simulink model "Drone2_simulink_old1"  (R2024b)
settings: Solver=ode1be  StartTime=0.0  StopTime=1200  FixedStep=0.001  MaxStep=0.001  MinStep=0.00095  RelTol=1e-3
undefined symbols (not defined in the file): DiscIntNeverNeededParam, Environment, Newton, Raphson, Sim3dSensor, Vehicle, X, Y, Z
libraries: sm_lib x2951, nesl_utility x76, slpidlib x25, simulink x4, eeGeneralControl x4, matrix_library x3, rllib x2, sim3dlib x2, uavsim3dlib x2, dspstat3 x1, SignalEditorBlockLib x1, sharedutil x1
(part 5 of 21)

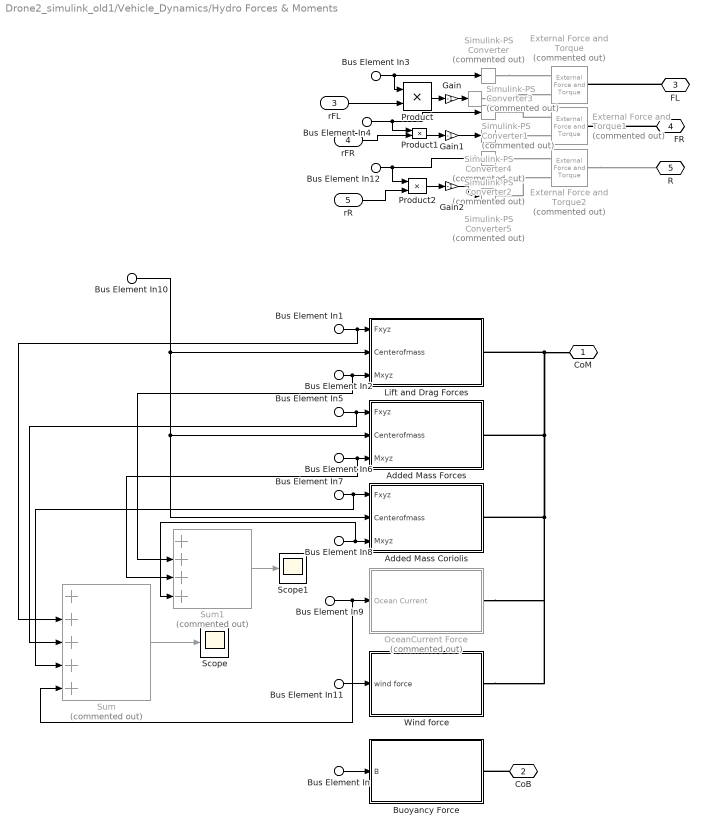
== system Drone2_simulink_old1/Vehicle_Dynamics/Hydro Forces & Moments ==
  Bus Element In1 : Inport  PortName=HydroForces  Element=Drag.Forces
  Bus Element In2 : Inport  PortName=HydroForces  Element=Drag.Moments
  Bus Element In : Inport  PortName=HydroForces  Element=BuoyancyForce
  Bus Element In5 : Inport  PortName=HydroForces  Element=AddedMass.AMForcesXYZ
  Bus Element In6 : Inport  PortName=HydroForces  Element=AddedMass.AMMomentsXYZ
  Bus Element In7 : Inport  PortName=HydroForces  Element=AddedMass.CForcesXYZ
  Bus Element In8 : Inport  PortName=HydroForces  Element=AddedMass.CMomentsXYZ
  Bus Element In9 : Inport  PortName=HydroForces  Element=OceanCurrentForce
  Bus Element In11 : Inport  PortName=HydroForces  Element=WindForce
  Bus Element In3 : Inport  PortName=HydroForces  Element=syringe.FL
  Bus Element In4 : Inport  PortName=HydroForces  Element=syringe.FR
  Bus Element In12 : Inport  PortName=HydroForces  Element=syringe.R
  Bus Element In10 : Inport  Port=2  PortName=CenterofMass  Element=Body.COM
  rFL : Inport  Port=3
  rFR : Inport  Port=4
  rR : Inport  Port=5
  Added Mass Coriolis : Subsystem
  Added Mass Forces : Subsystem
  Buoyancy Force : Subsystem
  External Force and Torque : sm_lib/Forces and Torques/External Force and Torque  Commented=on  EnableForceX=off  EnableForceY=off  EnableForceZ=on  EnableForce=off  ForceResolutionFrame=AttachedFrame  EnableTorqueX=off  EnableTorqueY=on  EnableTorqueZ=off  EnableTorque=off  TorqueResolutionFrame=AttachedFrame
  External Force and Torque1 : sm_lib/Forces and Torques/External Force and Torque  Commented=on  EnableForceX=off  EnableForceY=off  EnableForceZ=on  EnableForce=off  ForceResolutionFrame=AttachedFrame  EnableTorqueX=off  EnableTorqueY=on  EnableTorqueZ=off  EnableTorque=off  TorqueResolutionFrame=AttachedFrame
  External Force and Torque2 : sm_lib/Forces and Torques/External Force and Torque  Commented=on  EnableForceX=off  EnableForceY=off  EnableForceZ=on  EnableForce=off  ForceResolutionFrame=AttachedFrame  EnableTorqueX=off  EnableTorqueY=on  EnableTorqueZ=off  EnableTorque=off  TorqueResolutionFrame=AttachedFrame
  Gain : Gain  Gain=-1
  Gain1 : Gain  Gain=-1
  Gain2 : Gain  Gain=-1
  Lift and Drag Forces : Subsystem
  OceanCurrent Force : Subsystem  Commented=on
  Product : Product
  Product1 : Product
  Product2 : Product
  Scope : Scope
  Scope1 : Scope
  Simulink-PS Converter{,1..5} (6 alike) : nesl_utility/Simulink-PS Converter  Commented=on  PhysicalDomain=network_engine_domain  SubClassName=ps_input  LeftPortType=input  RightPortType=output  PseudoPeriodic=off  Frequencies=[]  NoiseDistribution=none  NoiseParameters=[]  Unit=1  AffineConversion=off  FilteringAndDerivatives=provide  SimscapeFilterOrder=1  InputFilterTimeConstant=0.001  UdotUserProvided=0
  Sum : Sum  Commented=on  Inputs=+++++
  Sum1 : Sum  Commented=on  Inputs=++++
  Wind force : Subsystem
  CoM : PMIOPort  Side=Left
  CoB : PMIOPort  Port=2  Side=Left
  FL : PMIOPort  Port=3  Side=Left
  FR : PMIOPort  Port=4  Side=Left
  R : PMIOPort  Port=5  Side=Left
  wires:
  Bus Element In/1 -> Buoyancy Force/1(B)
  Bus Element In1/1 -> Sum/2, Lift and Drag Forces/1(Fxyz)
  Bus Element In2/1 -> Sum1/2, Lift and Drag Forces/3(Mxyz)
  Bus Element In5/1 -> Sum/3, Added Mass Forces/1(Fxyz)
  Bus Element In8/1 -> Sum1/4, Added Mass Coriolis/3(Mxyz)
  Bus Element In9/1 -> Sum/5, OceanCurrent Force/1(Ocean Current)
  Bus Element In10/1 -> Lift and Drag Forces/2(Centerofmass), Added Mass Coriolis/2(Centerofmass), Added Mass Forces/2(Centerofmass)
  Bus Element In6/1 -> Sum1/3, Added Mass Forces/3(Mxyz)
  Bus Element In7/1 -> Sum/4, Added Mass Coriolis/1(Fxyz)
  Bus Element In11/1 -> Wind force/1(wind force)
  Sum/1 -> Scope/1
  Sum1/1 -> Scope1/1
  Bus Element In3/1 -> Product/1, Simulink-PS Converter/1
  Bus Element In4/1 -> Simulink-PS Converter1/1, Product1/1
  Product/1 -> Gain/1
  Gain1/1 -> Simulink-PS Converter4/1
  Gain2/1 -> Simulink-PS Converter5/1
  rFL/1 -> Product/2
  rFR/1 -> Product1/2
  Gain/1 -> Simulink-PS Converter3/1
  Product1/1 -> Gain1/1
  Bus Element In12/1 -> Product2/1, Simulink-PS Converter2/1
  rR/1 -> Product2/2
  Product2/1 -> Gain2/1
  connections:
  CoB/RConn1 -- Buoyancy Force/RConn1
  Wind force/RConn1 -- OceanCurrent Force/RConn1 -- Added Mass Coriolis/RConn1 -- Added Mass Forces/RConn1 -- CoM/RConn1 -- Lift and Drag Forces/RConn1
  Simulink-PS Converter/RConn1 -- External Force and Torque/LConn1
  External Force and Torque1/LConn1 -- Simulink-PS Converter1/RConn1
  Simulink-PS Converter2/RConn1 -- External Force and Torque2/LConn1
  FL/RConn1 -- External Force and Torque/RConn1
  FR/RConn1 -- External Force and Torque1/RConn1
  External Force and Torque2/RConn1 -- R/RConn1
  Simulink-PS Converter3/RConn1 -- External Force and Torque/LConn2
  Simulink-PS Converter4/RConn1 -- External Force and Torque1/LConn2
  Simulink-PS Converter5/RConn1 -- External Force and Torque2/LConn2

== system Drone2_simulink_old1/Vehicle_Dynamics/World ==
  Bottom floor : Subsystem  mask{ZB=-10, X=25, Z=0.1, Y=25, C1R=0.600, C1G=1, C1B=1.0, C2R=0, C2G=0.4, C2B=0.6}
      mask prompts: ZB "Distance of Bottom from World"; X "Length"; Z "Thikness"; Y "Width"; C1R "Red"; C1G "Green"; C1B "Blue"; C2R "Red"; C2G "Green"; C2B "Blue"
      mask init:
      | Color1 = [C1R C1G C1B];
      | Color2 = [C2R C2G C2B];
      mask DialogControl ParameterGroupVar Prompt: Bottom surface data
      mask DialogControl Container8 Prompt: Distance from World to Bottom
      mask DialogControl Container6 Prompt: Data of Each tiles
      mask DialogControl Container7 Prompt: Color 1
      mask DialogControl Container5 Prompt: Color2
      mask Display:
      | patch([0 10 10 0], [0 0 10 10], Color1);
      | patch([10 20 20 10], [0 0 10 10], Color2);
      | patch([0 10 10 0], [10 10 20 20], Color2);
      | patch([10 20 20 10], [10 10 20 20], Color1);
  Bottom floor1 : Subsystem  mask{ZB=-40, X=25, Z=0.1, Y=25, C1R=0.780, C1G=1.0, C1B=0.660, C2R=1.0, C2G=0.0, C2B=1.0}
      mask prompts: ZB "Distance of Bottom from World"; X "Length"; Z "Thikness"; Y "Width"; C1R "Red"; C1G "Green"; C1B "Blue"; C2R "Red"; C2G "Green"; C2B "Blue"
      mask init:
      | Color1 = [C1R C1G C1B];
      | Color2 = [C2R C2G C2B];
      mask DialogControl ParameterGroupVar Prompt: Bottom surface data
      mask DialogControl Container8 Prompt: Distance from World to Bottom
      mask DialogControl Container6 Prompt: Data of Each tiles
      mask DialogControl Container7 Prompt: Color 1
      mask DialogControl Container5 Prompt: Color2
      mask Display:
      | patch([0 10 10 0], [0 0 10 10], Color1);
      | patch([10 20 20 10], [0 0 10 10], Color2);
      | patch([0 10 10 0], [10 10 20 20], Color2);
      | patch([10 20 20 10], [10 10 20 20], Color1);
  Brick Solid : sm_lib/Body Elements/Brick Solid  Commented=on  BrickDimensions=[0.5 1 10]  BrickDimensionsUnits=m  ExportEntireGeometry=off  InertiaType=CalculateFromGeometry  BasedOnType=Density  Density=1000  DensityUnits=kg/m^3  Mass=1  MassUnits=kg  CenterOfMass=[0 0 0]  CenterOfMassUnits=m  MomentsOfInertia=[1 1 1]  MomentsOfInertiaUnits=kg*m^2  ProductsOfInertia=[0 0 0]  ProductsOfInertiaUnits=kg*m^2  GraphicType=FromGeometry  MarkerShape=Sphere  MarkerSize=10  GraphicVisPropType=SimpleVisualProperties  GraphicDiffuseColor=[1.0 0.2 0.2]  GraphicOpacity=1  GraphicSpecularColor=[0.5 0.5 0.5 1.0]  GraphicAmbientColor=[0.15 0.15 0.15 1.0]  GraphicEmissiveColor=[0.0 0.0 0.0 1.0]  GraphicShininess=75  DoExposeReferenceFrame=on  SerializedFrames=<Frames/>
  Brick Solid1 : sm_lib/Body Elements/Brick Solid  Commented=on  BrickDimensions=[0.5 1 10]  BrickDimensionsUnits=m  ExportEntireGeometry=off  InertiaType=CalculateFromGeometry  BasedOnType=Density  Density=1000  DensityUnits=kg/m^3  Mass=1  MassUnits=kg  CenterOfMass=[0 0 0]  CenterOfMassUnits=m  MomentsOfInertia=[1 1 1]  MomentsOfInertiaUnits=kg*m^2  ProductsOfInertia=[0 0 0]  ProductsOfInertiaUnits=kg*m^2  GraphicType=FromGeometry  MarkerShape=Sphere  MarkerSize=10  GraphicVisPropType=SimpleVisualProperties  GraphicDiffuseColor=[1.0 0.2 0.2]  GraphicOpacity=1  GraphicSpecularColor=[0.5 0.5 0.5 1.0]  GraphicAmbientColor=[0.15 0.15 0.15 1.0]  GraphicEmissiveColor=[0.0 0.0 0.0 1.0]  GraphicShininess=75  DoExposeReferenceFrame=on  SerializedFrames=<Frames/>
  MechanismConfiguration : sm_lib/Utilities/Mechanism Configuration  UniformGravity=Constant  GravityVector=[0 0 Environment.gravity]  GravityVectorUnits=m/s^2  LinearizationDelta=0.001  JointModeTransitionNonlinearIterations=2
  Solver Configuration : nesl_utility/Solver Configuration  PhysicalDomain=network_engine_domain  SubClassName=solver  LeftPortType=input  RightPortType=generic  Tones=[]  Harmonics=[]  SimulateNoise=off  Profile=off  UseLocalSampling=off  EnableSwitchedLinearOptims=on  FrequencyDomain=off  UseCCode=off  RelTol=0.001  AbsTol=0.001  MinStep=1e-09  ToWorkspace=off  RevertToSquareIcSolve=off  NumHomotopyIterations=100  PhasorMode=off  PhasorModeNumHarmonics=1  ConsistencySolver=NEWTON_XTOL_AFTER_FTOL  IndexReductionMethod=DerivativeReplacement  DoDC=off  ResidualTolerance=1e-09  ConsistencyTolSource=LOCAL  ConsistencyAbsTol=0.001  ConsistencyRelTol=0.001  ConsistencyTolFactor=0.001  UseLocalSolver=on  LocalSolverChoice=NE_BACKWARD_EULER_ADVANCER  ResolveIndetEquations=on  FunctionEvalNumThread=1  LocalSolverSampleTime=0.001  DoFixedCost=on  MaxNonlinIter=3  MaxModeIter=2  ComputeImpulses=off  ImpulseIterations=2  LinearAlgebra=Sparse  LinearAlgebraNumThread=0  EquationFormulation=NE_TIME_EF  DelaysMemoryBudget=1024  AutomaticFiltering=off  FilteringTimeConstant=0.001  PartitionStorageMethod=AS_NEEDED  PartitionMemoryBudget=1024  PartitionMethod=ROBUST  MultibodyUseLocalSolver=off  MultibodyLocalSolverChoice=ODE4  MultibodyLocalSolverSampleTime=0.001
  Spatial Contact Force : sm_lib/Forces and Torques/Spatial Contact Force  NormalForceType=SmoothSpringDamper  NormalStiffness=1  NormalStiffnessUnits=N/m  NormalDamping=0.001  NormalDampingUnits=N/(m/s)  NormalTransitionRegionWidth=0.05  NormalTransitionRegionWidthUnits=m  FrictionType=None  CoefficientOfStaticFriction=0  CoefficientOfDynamicFriction=0  FrictionalCriticalVelocity=1  FrictionalCriticalVelocityUnits=m/s  SenseContactSignal=off  SensePenetrationDepth=off  SenseSeparationDistance=off  SenseNormalForceMagnitude=off  SenseFrictionalForceMagnitude=off  SenseNormalVelocity=off  SenseTangentialVelocity=off  SenseContactBaseRotation=off  SenseContactBaseTranslation=off  SenseContactFollowerRotation=off  SenseContactFollowerTranslation=off  ZeroCrossDetectContactStartAndEnd=off
  Spatial Contact Force1 : sm_lib/Forces and Torques/Spatial Contact Force  NormalForceType=SmoothSpringDamper  NormalStiffness=1e2  NormalStiffnessUnits=N/m  NormalDamping=1e3  NormalDampingUnits=N/(m/s)  NormalTransitionRegionWidth=1e-4  NormalTransitionRegionWidthUnits=m  FrictionType=SmoothStickSlip  CoefficientOfStaticFriction=0.5  CoefficientOfDynamicFriction=0.3  FrictionalCriticalVelocity=1e-3  FrictionalCriticalVelocityUnits=m/s  SenseContactSignal=off  SensePenetrationDepth=off  SenseSeparationDistance=off  SenseNormalForceMagnitude=off  SenseFrictionalForceMagnitude=off  SenseNormalVelocity=off  SenseTangentialVelocity=off  SenseContactBaseRotation=off  SenseContactBaseTranslation=off  SenseContactFollowerRotation=off  SenseContactFollowerTranslation=off  ZeroCrossDetectContactStartAndEnd=off
  World : sm_lib/Frames and Transforms/World Frame
  water surface : sm_lib/Body Elements/Brick Solid  BrickDimensions=[500 500 0.01]  BrickDimensionsUnits=m  ExportEntireGeometry=on  InertiaType=CalculateFromGeometry  BasedOnType=Density  Density=1  DensityUnits=kg/m^3  Mass=1  MassUnits=kg  CenterOfMass=[0 0 0]  CenterOfMassUnits=m  MomentsOfInertia=[1 1 1]  MomentsOfInertiaUnits=kg*m^2  ProductsOfInertia=[0 0 0]  ProductsOfInertiaUnits=kg*m^2  GraphicType=FromGeometry  MarkerShape=Sphere  MarkerSize=10  GraphicVisPropType=SimpleVisualProperties  GraphicDiffuseColor=[0.0 0.8 1.0]  GraphicOpacity=0.1  GraphicSpecularColor=[0.5 0.5 0.5 1.0]  GraphicAmbientColor=[0.15 0.15 0.15 1.0]  GraphicEmissiveColor=[0.0 0.0 0.0 1.0]  GraphicShininess=75  DoExposeReferenceFrame=on  SerializedFrames=<Frames/>
  water surface ti bottom : sm_lib/Frames and Transforms/Rigid Transform  RotationMethod=None  FollAlignAxisA=+X  BaseAlignAxisA=+Y  FollAlignAxisB=+Y  BaseAlignAxisB=+Z  RotationStandardAxis=+Z  RotationAngle=0  RotationAngleUnits=deg  RotationArbitraryAxis=[0 0 1]  RotationSequenceAxes=FollowerAxes  RotationSequence=XYX  RotationSequenceAngles=[0 0 0]  RotationSequenceAnglesUnits=deg  RotationMatrix=[1 0 0;0 1 0;0 0 1]  Quaternion=[1 0 0 0]  TranslationMethod=Cartesian  TranslationCartesianOffset=[0 0 0]  TranslationCartesianOffsetUnits=m  TranslationStandardAxis=+Z  TranslationStandardOffset=0  TranslationStandardOffsetUnits=m  TranslationROffset=0  TranslationROffsetUnits=m  TranslationThetaOffset=0  TranslationThetaOffsetUnits=deg  TranslationZOffset=0  TranslationZOffsetUnits=m
  water surface ti bottom1 : sm_lib/Frames and Transforms/Rigid Transform  Commented=on  RotationMethod=None  FollAlignAxisA=+X  BaseAlignAxisA=+Y  FollAlignAxisB=+Y  BaseAlignAxisB=+Z  RotationStandardAxis=+Z  RotationAngle=0  RotationAngleUnits=deg  RotationArbitraryAxis=[0 0 1]  RotationSequenceAxes=FollowerAxes  RotationSequence=XYX  RotationSequenceAngles=[0 0 0]  RotationSequenceAnglesUnits=deg  RotationMatrix=[1 0 0;0 1 0;0 0 1]  Quaternion=[1 0 0 0]  TranslationMethod=Cartesian  TranslationCartesianOffset=[25 0 -5]  TranslationCartesianOffsetUnits=m  TranslationStandardAxis=+Z  TranslationStandardOffset=0  TranslationStandardOffsetUnits=m  TranslationROffset=0  TranslationROffsetUnits=m  TranslationThetaOffset=0  TranslationThetaOffsetUnits=deg  TranslationZOffset=0  TranslationZOffsetUnits=m
  water surface ti bottom2 : sm_lib/Frames and Transforms/Rigid Transform  Commented=on  RotationMethod=None  FollAlignAxisA=+X  BaseAlignAxisA=+Y  FollAlignAxisB=+Y  BaseAlignAxisB=+Z  RotationStandardAxis=+Z  RotationAngle=0  RotationAngleUnits=deg  RotationArbitraryAxis=[0 0 1]  RotationSequenceAxes=FollowerAxes  RotationSequence=XYX  RotationSequenceAngles=[0 0 0]  RotationSequenceAnglesUnits=deg  RotationMatrix=[1 0 0;0 1 0;0 0 1]  Quaternion=[1 0 0 0]  TranslationMethod=Cartesian  TranslationCartesianOffset=[10 15 -5]  TranslationCartesianOffsetUnits=m  TranslationStandardAxis=+Z  TranslationStandardOffset=0  TranslationStandardOffsetUnits=m  TranslationROffset=0  TranslationROffsetUnits=m  TranslationThetaOffset=0  TranslationThetaOffsetUnits=deg  TranslationZOffset=0  TranslationZOffsetUnits=m
  water surface ti bottom3 : sm_lib/Frames and Transforms/Rigid Transform  RotationMethod=AlignedAxes  FollAlignAxisA=+X  BaseAlignAxisA=+X  FollAlignAxisB=-Z  BaseAlignAxisB=+Y  RotationStandardAxis=+Z  RotationAngle=0  RotationAngleUnits=deg  RotationArbitraryAxis=[0 0 1]  RotationSequenceAxes=FollowerAxes  RotationSequence=XYX  RotationSequenceAngles=[0 0 0]  RotationSequenceAnglesUnits=deg  RotationMatrix=[1 0 0;0 1 0;0 0 1]  Quaternion=[1 0 0 0]  TranslationMethod=Cartesian  TranslationCartesianOffset=[0 0 0]  TranslationCartesianOffsetUnits=m  TranslationStandardAxis=+Z  TranslationStandardOffset=0  TranslationStandardOffsetUnits=m  TranslationROffset=0  TranslationROffsetUnits=m  TranslationThetaOffset=0  TranslationThetaOffsetUnits=deg  TranslationZOffset=0  TranslationZOffsetUnits=m
  surface : PMIOPort  Side=Right
  bottomsurf : PMIOPort  Port=2  Side=Right
  W : PMIOPort  Port=3  Side=Right
  connections:
  water surface/LConn1 -- Spatial Contact Force/LConn1
  surface/RConn1 -- Spatial Contact Force/RConn1
  bottomsurf/RConn1 -- Spatial Contact Force1/RConn1
  World/RConn1 -- water surface ti bottom3/LConn1 -- water surface ti bottom1/LConn1 -- water surface ti bottom2/LConn1 -- Solver Configuration/RConn1 -- water surface ti bottom/LConn1 -- water surface/RConn1 -- MechanismConfiguration/RConn1 -- W/RConn1
  Bottom floor/LConn1 -- water surface ti bottom/RConn1
  Bottom floor/RConn1 -- Spatial Contact Force1/LConn1
  Brick Solid/RConn1 -- water surface ti bottom1/RConn1
  Brick Solid1/RConn1 -- water surface ti bottom2/RConn1
  Bottom floor1/LConn1 -- water surface ti bottom3/RConn1

== system Drone2_simulink_old1/Visualization/psidot ==
  pqr : Inport
  phithetapsi : Inport  Port=2
  Mux1 : Mux  Inputs=[3 3 3]
  psidot : Fcn  Expr=(u[2]*u[4]+u[3]*u[7])/u[8]
  sincos : Trigonometry  Operator=sincos
  psid : Outport  Unit=rad/s  InitialOutput=0  VectorParamsAs1DForOutWhenUnconnected=off
  wires:
  sincos/2 -> Mux1/3
  sincos/1 -> Mux1/2
  phithetapsi/1 -> sincos/1
  pqr/1 -> Mux1/1
  Mux1/1 -> psidot/1
  psidot/1 -> psid/1

== system Drone2_simulink_old1/Controller (STA-Based)/Subsystem1/norm force ==
  force : Inport
  Add : Sum
  Add2 : Sum  Inputs=|++
  Demux2 : Demux  Outputs=2
  Gain : Gain  Gain=2
  Gain1 : Gain  Gain=2
  Sqrt : Sqrt
  Square : Math  Operator=square
  Square1 : Math  Operator=square
  Terminator : Terminator
  sum : Outport
  wires:
  Square1/1 -> Add/2
  Add/1 -> Sqrt/1
  Demux2/1 -> Gain1/1, Square/1
  Demux2/2 -> Add2/2, Square1/1
  Square/1 -> Gain/1
  force/1 -> Demux2/1
  Gain/1 -> Add/1
  Gain1/1 -> Add2/1
  Add2/1 -> sum/1
  Sqrt/1 -> Terminator/1  "norm"

== system Drone2_simulink_old1/Drive Controls/Thrust Controls/Depth and Pitch Control ==
  note: NOTE: Vehicle depth is indirectly controlled by the pitch angle which is regulated by the vertical thrusters ONLY
  PPf : Inport
  SPf : Inport  Port=2
  ZRef : Inport  Port=3
  Z : Inport  Port=4
  theta : Inport  Port=5
  Gain2 : Gain  Gain=-1
  Main Propellers Thrust Offset Compensation : Subsystem
  PDtheta : slpidlib/PID Controller  Controller=PD  Form=Parallel  TimeDomain=Continuous-time  UseExternalTs=off  SampleTime=-1  IntegratorMethod=Forward Euler  FilterMethod=Forward Euler  ControllerParametersSource=internal  P=-2023.58  I=1  UseKiTs=off  D=-2454.43  UseExternalDerivativeSource=off  N=3588.47  UseFilter=on  TunerSelectOption=Transfer Function Based (PID Tuner App)  InitialConditionSource=internal  InitialConditionForIntegrator=0  InitialConditionForFilter=0  DifferentiatorICPrevScaledInput=0  ExternalReset=none  TrackingMode=off  Kt=1  LimitOutput=off  SatLimitsSource=internal  UpperSaturationLimit=inf  LowerSaturationLimit=-inf  LinearizeAsGain=on  AntiWindupMode=none  Kb=1  LimitIntegrator=off  UpperIntegratorSaturationLimit=inf  LowerIntegratorSaturationLimit=-inf  POutMin=[]  POutMax=[]  IOutMin=[]  IOutMax=[]  DOutMin=[]  DOutMax=[]  NOutMin=[]  NOutMax=[]  SumOutMin=[]  SumOutMax=[]  SaturationOutMin=[]  SaturationOutMax=[]  PParamMin=[]  PParamMax=[]  IParamMin=[]  IParamMax=[]  DParamMin=[]  DParamMax=[]  NParamMin=[]  NParamMax=[]  KbParamMin=[]  KbParamMax=[]  KtParamMin=[]  KtParamMax=[]  KbOutMin=[]  KbOutMax=[]  KtOutMin=[]  KtOutMax=[]  IntegratorOutMin=[]  IntegratorOutMax=[]  FilterOutMin=[]  FilterOutMax=[]  SumI1OutMin=[]  SumI1OutMax=[]  SumI2OutMin=[]  SumI2OutMax=[]  SumI3OutMin=[]  SumI3OutMax=[]  SumI4OutMin=[]  SumI4OutMax=[]  SumDOutMin=[]  SumDOutMax=[]  DifferentiatorOutMin=[]  DifferentiatorOutMax=[]  FilterDiffOutCoefMin=[]  FilterDiffOutCoefMax=[]  ReciprocalOutMin=[]  ReciprocalOutMax=[]  SumDenOutMin=[]  SumDenOutMax=[]  SumNumOutMin=[]  SumNumOutMax=[]  DivideOutMin=[]  DivideOutMax=[]  UdiffTsProdOutMin=[]  UdiffTsProdOutMax=[]  NTsProdOutMin=[]  NTsProdOutMax=[]  UintegralTsProdOutMin=[]  UintegralTsProdOutMax=[]  UngainTsProdOutMin=[]  UngainTsProdOutMax=[]  ClampingZeroOutDataTypeStr=Inherit: Inherit via back propagation  ClampingZeroOutMin=[]  ClampingZeroOutMax=[]  FilterDenConstantOutDataTypeStr=Inherit: Inherit via back propagation  FilterDenConstantOutMin=[]  FilterDenConstantOutMax=[]  PCopyOutDataTypeStr=Inherit: Inherit via back propagation  PCopyOutMin=[]  PCopyOutMax=[]  NCopyOutDataTypeStr=Inherit: Inherit via back propagation  NCopyOutMin=[]  NCopyOutMax=[]  IntegratorContinuousStateAttributes=''  IntegratorStateMustResolveToSignalObject=off  IntegratorRTWStateStorageClass=Auto  FilterContinuousStateAttributes=''  FilterStateMustResolveToSignalObject=off  FilterRTWStateStorageClass=Auto  ParallelPVariant=InternalParameters  IdealPVariant=Disabled  IVariant=Disabled  DVariant=InternalParameters  IntegratorVariant=Disabled  SatVariant=Disabled  AWVariant=Disabled  PCopyVariant=Disabled  TRVariant=Disabled  FdbkBlocksVariant=Forward  IdealPFdbkVariant=Disabled  SatFdbkVariant=Disabled  DerivativeFilterVariant=ContFilter  NVariant=InternalParameters  NCopyVariant=Disabled  FilterICVariant=InternalICsFilter  IntegratorICVariant=Disabled  ExternalResetVariant=Disabled  TRSumVariant=Passthrough  SumFdbkVariant=Disabled  SumVariant=Sum_PD  TsampFilterVariant=InternalTs  TsampNgainVariant=Passthrough  TsampIntegralVariant=Disabled_SignalSpec  ExternalSaturationOutDataTypeStr=Inherit: Same as second input  DerivativeSourceVariant=ErrorSignal
  PIZ : slpidlib/PID Controller  Controller=PI  Form=Parallel  TimeDomain=Continuous-time  UseExternalTs=off  SampleTime=-1  IntegratorMethod=Forward Euler  FilterMethod=Forward Euler  ControllerParametersSource=internal  P=-0.25  I=-0.001  UseKiTs=off  D=0  UseExternalDerivativeSource=off  N=100  UseFilter=on  TunerSelectOption=Transfer Function Based (PID Tuner App)  InitialConditionSource=internal  InitialConditionForIntegrator=0  InitialConditionForFilter=0  DifferentiatorICPrevScaledInput=0  ExternalReset=none  TrackingMode=off  Kt=1  LimitOutput=off  SatLimitsSource=internal  UpperSaturationLimit=inf  LowerSaturationLimit=-inf  LinearizeAsGain=on  AntiWindupMode=none  Kb=1  LimitIntegrator=off  UpperIntegratorSaturationLimit=inf  LowerIntegratorSaturationLimit=-inf  POutMin=[]  POutMax=[]  IOutMin=[]  IOutMax=[]  DOutMin=[]  DOutMax=[]  NOutMin=[]  NOutMax=[]  SumOutMin=[]  SumOutMax=[]  SaturationOutMin=[]  SaturationOutMax=[]  PParamMin=[]  PParamMax=[]  IParamMin=[]  IParamMax=[]  DParamMin=[]  DParamMax=[]  NParamMin=[]  NParamMax=[]  KbParamMin=[]  KbParamMax=[]  KtParamMin=[]  KtParamMax=[]  KbOutMin=[]  KbOutMax=[]  KtOutMin=[]  KtOutMax=[]  IntegratorOutMin=[]  IntegratorOutMax=[]  FilterOutMin=[]  FilterOutMax=[]  SumI1OutMin=[]  SumI1OutMax=[]  SumI2OutMin=[]  SumI2OutMax=[]  SumI3OutMin=[]  SumI3OutMax=[]  SumI4OutMin=[]  SumI4OutMax=[]  SumDOutMin=[]  SumDOutMax=[]  DifferentiatorOutMin=[]  DifferentiatorOutMax=[]  FilterDiffOutCoefMin=[]  FilterDiffOutCoefMax=[]  ReciprocalOutMin=[]  ReciprocalOutMax=[]  SumDenOutMin=[]  SumDenOutMax=[]  SumNumOutMin=[]  SumNumOutMax=[]  DivideOutMin=[]  DivideOutMax=[]  UdiffTsProdOutMin=[]  UdiffTsProdOutMax=[]  NTsProdOutMin=[]  NTsProdOutMax=[]  UintegralTsProdOutMin=[]  UintegralTsProdOutMax=[]  UngainTsProdOutMin=[]  UngainTsProdOutMax=[]  ClampingZeroOutDataTypeStr=Inherit: Inherit via back propagation  ClampingZeroOutMin=[]  ClampingZeroOutMax=[]  FilterDenConstantOutDataTypeStr=Inherit: Inherit via back propagation  FilterDenConstantOutMin=[]  FilterDenConstantOutMax=[]  PCopyOutDataTypeStr=Inherit: Inherit via back propagation  PCopyOutMin=[]  PCopyOutMax=[]  NCopyOutDataTypeStr=Inherit: Inherit via back propagation  NCopyOutMin=[]  NCopyOutMax=[]  IntegratorContinuousStateAttributes=''  IntegratorStateMustResolveToSignalObject=off  IntegratorRTWStateStorageClass=Auto  FilterContinuousStateAttributes=''  FilterStateMustResolveToSignalObject=off  FilterRTWStateStorageClass=Auto  ParallelPVariant=InternalParameters  IdealPVariant=Disabled  IVariant=InternalParameters  DVariant=Disabled  IntegratorVariant=Continuous  SatVariant=Disabled  AWVariant=Passthrough  PCopyVariant=Disabled  TRVariant=Disabled  FdbkBlocksVariant=Forward  IdealPFdbkVariant=Disabled  SatFdbkVariant=Disabled  DerivativeFilterVariant=Disabled  NVariant=Disabled  NCopyVariant=Disabled_SignalSpec  FilterICVariant=Disabled  IntegratorICVariant=InternalICs  ExternalResetVariant=Disabled  TRSumVariant=Passthrough  SumFdbkVariant=Disabled  SumVariant=Sum_PI  TsampFilterVariant=InternalTs  TsampNgainVariant=Passthrough  TsampIntegralVariant=Disabled_SignalSpec  ExternalSaturationOutDataTypeStr=Inherit: Same as second input  DerivativeSourceVariant=Disabled
  Sum : Sum  Inputs=|+-
  Sum1 : Sum  Inputs=++|
  Sum2 : Sum  Inputs=|+-
  BVTfcmd : Outport
  SVTfcmd : Outport  Port=2
  wires:
  PPf/1 -> Main Propellers Thrust Offset Compensation/1(PPf)
  SPf/1 -> Main Propellers Thrust Offset Compensation/2(SPf)
  Gain2/1 -> SVTfcmd/1
  theta/1 -> Sum/2
  Sum/1 -> PDtheta/1
  PDtheta/1 -> Sum1/2
  Sum1/1 -> Gain2/1, BVTfcmd/1
  ZRef/1 -> Sum2/1
  Z/1 -> Sum2/2
  Sum2/1 -> PIZ/1
  PIZ/1 -> Sum/1
  Main Propellers Thrust Offset Compensation/1(VTf) -> Sum1/1

== system Drone2_simulink_old1/Drive Controls/Thrust Controls/Heading and Yaw Control ==
  note: NOTE: Vehicle heading is regulated by the horizontal thrusters ONLY
  v : Inport
  psiRef : Inport  Port=2
  pqr : Inport  Port=3
  phithetapsi : Inport  Port=4
  Bus Selector : BusSelector  OutputSignals=psi
  Gain : Gain  Gain=-1
  PIDpsi : slpidlib/PID Controller  Controller=PID  Form=Parallel  TimeDomain=Continuous-time  UseExternalTs=off  SampleTime=-1  IntegratorMethod=Forward Euler  FilterMethod=Forward Euler  ControllerParametersSource=internal  P=564.0086345182  I=63718.733398644  UseKiTs=off  D=1.06148768314347  UseExternalDerivativeSource=off  N=71769.5968954127  UseFilter=on  TunerSelectOption=Transfer Function Based (PID Tuner App)  InitialConditionSource=internal  InitialConditionForIntegrator=0  InitialConditionForFilter=0  DifferentiatorICPrevScaledInput=0  ExternalReset=none  TrackingMode=off  Kt=1  LimitOutput=off  SatLimitsSource=internal  UpperSaturationLimit=inf  LowerSaturationLimit=-inf  LinearizeAsGain=on  AntiWindupMode=none  Kb=1  LimitIntegrator=off  UpperIntegratorSaturationLimit=inf  LowerIntegratorSaturationLimit=-inf  POutMin=[]  POutMax=[]  IOutMin=[]  IOutMax=[]  DOutMin=[]  DOutMax=[]  NOutMin=[]  NOutMax=[]  SumOutMin=[]  SumOutMax=[]  SaturationOutMin=[]  SaturationOutMax=[]  PParamMin=[]  PParamMax=[]  IParamMin=[]  IParamMax=[]  DParamMin=[]  DParamMax=[]  NParamMin=[]  NParamMax=[]  KbParamMin=[]  KbParamMax=[]  KtParamMin=[]  KtParamMax=[]  KbOutMin=[]  KbOutMax=[]  KtOutMin=[]  KtOutMax=[]  IntegratorOutMin=[]  IntegratorOutMax=[]  FilterOutMin=[]  FilterOutMax=[]  SumI1OutMin=[]  SumI1OutMax=[]  SumI2OutMin=[]  SumI2OutMax=[]  SumI3OutMin=[]  SumI3OutMax=[]  SumI4OutMin=[]  SumI4OutMax=[]  SumDOutMin=[]  SumDOutMax=[]  DifferentiatorOutMin=[]  DifferentiatorOutMax=[]  FilterDiffOutCoefMin=[]  FilterDiffOutCoefMax=[]  ReciprocalOutMin=[]  ReciprocalOutMax=[]  SumDenOutMin=[]  SumDenOutMax=[]  SumNumOutMin=[]  SumNumOutMax=[]  DivideOutMin=[]  DivideOutMax=[]  UdiffTsProdOutMin=[]  UdiffTsProdOutMax=[]  NTsProdOutMin=[]  NTsProdOutMax=[]  UintegralTsProdOutMin=[]  UintegralTsProdOutMax=[]  UngainTsProdOutMin=[]  UngainTsProdOutMax=[]  ClampingZeroOutDataTypeStr=Inherit: Inherit via back propagation  ClampingZeroOutMin=[]  ClampingZeroOutMax=[]  FilterDenConstantOutDataTypeStr=Inherit: Inherit via back propagation  FilterDenConstantOutMin=[]  FilterDenConstantOutMax=[]  PCopyOutDataTypeStr=Inherit: Inherit via back propagation  PCopyOutMin=[]  PCopyOutMax=[]  NCopyOutDataTypeStr=Inherit: Inherit via back propagation  NCopyOutMin=[]  NCopyOutMax=[]  IntegratorContinuousStateAttributes=''  IntegratorStateMustResolveToSignalObject=off  IntegratorRTWStateStorageClass=Auto  FilterContinuousStateAttributes=''  FilterStateMustResolveToSignalObject=off  FilterRTWStateStorageClass=Auto  ParallelPVariant=InternalParameters  IdealPVariant=Disabled  IVariant=InternalParameters  DVariant=InternalParameters  IntegratorVariant=Continuous  SatVariant=Disabled  AWVariant=Passthrough  PCopyVariant=Disabled  TRVariant=Disabled  FdbkBlocksVariant=Forward  IdealPFdbkVariant=Disabled  SatFdbkVariant=Disabled  DerivativeFilterVariant=ContFilter  NVariant=InternalParameters  NCopyVariant=Disabled  FilterICVariant=InternalICsFilter  IntegratorICVariant=InternalICs  ExternalResetVariant=Disabled  TRSumVariant=Passthrough  SumFdbkVariant=Disabled  SumVariant=Sum_PID  TsampFilterVariant=InternalTs  TsampNgainVariant=Passthrough  TsampIntegralVariant=Disabled_SignalSpec  ExternalSaturationOutDataTypeStr=Inherit: Same as second input  DerivativeSourceVariant=ErrorSignal
  PIDpsidot : slpidlib/PID Controller  Controller=PID  Form=Parallel  TimeDomain=Continuous-time  UseExternalTs=off  SampleTime=-1  IntegratorMethod=Forward Euler  FilterMethod=Forward Euler  ControllerParametersSource=internal  P=36876.176480623  I=4618545.3057506  UseKiTs=off  D=-22.9389890340326  UseExternalDerivativeSource=off  N=628  UseFilter=on  TunerSelectOption=Transfer Function Based (PID Tuner App)  InitialConditionSource=internal  InitialConditionForIntegrator=0  InitialConditionForFilter=0  DifferentiatorICPrevScaledInput=0  ExternalReset=none  TrackingMode=off  Kt=1  LimitOutput=off  SatLimitsSource=internal  UpperSaturationLimit=inf  LowerSaturationLimit=-inf  LinearizeAsGain=on  AntiWindupMode=none  Kb=1  LimitIntegrator=off  UpperIntegratorSaturationLimit=inf  LowerIntegratorSaturationLimit=-inf  POutMin=[]  POutMax=[]  IOutMin=[]  IOutMax=[]  DOutMin=[]  DOutMax=[]  NOutMin=[]  NOutMax=[]  SumOutMin=[]  SumOutMax=[]  SaturationOutMin=[]  SaturationOutMax=[]  PParamMin=[]  PParamMax=[]  IParamMin=[]  IParamMax=[]  DParamMin=[]  DParamMax=[]  NParamMin=[]  NParamMax=[]  KbParamMin=[]  KbParamMax=[]  KtParamMin=[]  KtParamMax=[]  KbOutMin=[]  KbOutMax=[]  KtOutMin=[]  KtOutMax=[]  IntegratorOutMin=[]  IntegratorOutMax=[]  FilterOutMin=[]  FilterOutMax=[]  SumI1OutMin=[]  SumI1OutMax=[]  SumI2OutMin=[]  SumI2OutMax=[]  SumI3OutMin=[]  SumI3OutMax=[]  SumI4OutMin=[]  SumI4OutMax=[]  SumDOutMin=[]  SumDOutMax=[]  DifferentiatorOutMin=[]  DifferentiatorOutMax=[]  FilterDiffOutCoefMin=[]  FilterDiffOutCoefMax=[]  ReciprocalOutMin=[]  ReciprocalOutMax=[]  SumDenOutMin=[]  SumDenOutMax=[]  SumNumOutMin=[]  SumNumOutMax=[]  DivideOutMin=[]  DivideOutMax=[]  UdiffTsProdOutMin=[]  UdiffTsProdOutMax=[]  NTsProdOutMin=[]  NTsProdOutMax=[]  UintegralTsProdOutMin=[]  UintegralTsProdOutMax=[]  UngainTsProdOutMin=[]  UngainTsProdOutMax=[]  ClampingZeroOutDataTypeStr=Inherit: Inherit via back propagation  ClampingZeroOutMin=[]  ClampingZeroOutMax=[]  FilterDenConstantOutDataTypeStr=Inherit: Inherit via back propagation  FilterDenConstantOutMin=[]  FilterDenConstantOutMax=[]  PCopyOutDataTypeStr=Inherit: Inherit via back propagation  PCopyOutMin=[]  PCopyOutMax=[]  NCopyOutDataTypeStr=Inherit: Inherit via back propagation  NCopyOutMin=[]  NCopyOutMax=[]  IntegratorContinuousStateAttributes=''  IntegratorStateMustResolveToSignalObject=off  IntegratorRTWStateStorageClass=Auto  FilterContinuousStateAttributes=''  FilterStateMustResolveToSignalObject=off  FilterRTWStateStorageClass=Auto  ParallelPVariant=InternalParameters  IdealPVariant=Disabled  IVariant=InternalParameters  DVariant=InternalParameters  IntegratorVariant=Continuous  SatVariant=Disabled  AWVariant=Passthrough  PCopyVariant=Disabled  TRVariant=Disabled  FdbkBlocksVariant=Forward  IdealPFdbkVariant=Disabled  SatFdbkVariant=Disabled  DerivativeFilterVariant=ContFilter  NVariant=InternalParameters  NCopyVariant=Disabled  FilterICVariant=InternalICsFilter  IntegratorICVariant=InternalICs  ExternalResetVariant=Disabled  TRSumVariant=Passthrough  SumFdbkVariant=Disabled  SumVariant=Sum_PID  TsampFilterVariant=InternalTs  TsampNgainVariant=Passthrough  TsampIntegralVariant=Disabled_SignalSpec  ExternalSaturationOutDataTypeStr=Inherit: Same as second input  DerivativeSourceVariant=ErrorSignal
  Sum : Sum  Inputs=-+|
  Sum1 : Sum  Inputs=-+|
  Sum2 : Sum  Inputs=++|
  Sum3 : Sum  Inputs=++|
  psidot : Subsystem
  side slip compensation : Subsystem
  BHTfcmd : Outport
  SHTfcmd : Outport  Port=2
  wires:
  pqr/1 -> psidot/1(pqr)
  phithetapsi/1 -> psidot/2(phithetapsi), Bus Selector/1
  psidot/1(psid) -> Sum/1
  Sum/1 -> PIDpsidot/1
  PIDpsidot/1 -> Gain/1, Sum2/2
  Sum1/1 -> PIDpsi/1
  PIDpsi/1 -> Sum/2
  Bus Selector/1 -> Sum1/1  "<psi>"
  psiRef/1 -> Sum1/2
  Sum2/1 -> BHTfcmd/1
  Gain/1 -> Sum3/2
  Sum3/1 -> SHTfcmd/1
  v/1 -> side slip compensation/1(v)
  side slip compensation/1(BHTf) -> Sum2/1
  side slip compensation/2(SHTf) -> Sum3/1

== system Drone2_simulink_old1/Drive Controls/Thrust Controls/Longitudinal Speed (Surge) Control ==
  note: NOTE: Vehicle longitudinal speed is regulated by the main propellers ONLY
  uRef : Inport
  u : Inport  Port=2
  PIu : slpidlib/PID Controller  Controller=PI  Form=Parallel  TimeDomain=Continuous-time  UseExternalTs=off  SampleTime=-1  IntegratorMethod=Forward Euler  FilterMethod=Forward Euler  ControllerParametersSource=internal  P=78.8975  I=17.2606  UseKiTs=off  D=0  UseExternalDerivativeSource=off  N=100  UseFilter=on  TunerSelectOption=Transfer Function Based (PID Tuner App)  InitialConditionSource=internal  InitialConditionForIntegrator=0  InitialConditionForFilter=0  DifferentiatorICPrevScaledInput=0  ExternalReset=none  TrackingMode=off  Kt=1  LimitOutput=off  SatLimitsSource=internal  UpperSaturationLimit=inf  LowerSaturationLimit=-inf  LinearizeAsGain=on  AntiWindupMode=none  Kb=1  LimitIntegrator=off  UpperIntegratorSaturationLimit=inf  LowerIntegratorSaturationLimit=-inf  POutMin=[]  POutMax=[]  IOutMin=[]  IOutMax=[]  DOutMin=[]  DOutMax=[]  NOutMin=[]  NOutMax=[]  SumOutMin=[]  SumOutMax=[]  SaturationOutMin=[]  SaturationOutMax=[]  PParamMin=[]  PParamMax=[]  IParamMin=[]  IParamMax=[]  DParamMin=[]  DParamMax=[]  NParamMin=[]  NParamMax=[]  KbParamMin=[]  KbParamMax=[]  KtParamMin=[]  KtParamMax=[]  KbOutMin=[]  KbOutMax=[]  KtOutMin=[]  KtOutMax=[]  IntegratorOutMin=[]  IntegratorOutMax=[]  FilterOutMin=[]  FilterOutMax=[]  SumI1OutMin=[]  SumI1OutMax=[]  SumI2OutMin=[]  SumI2OutMax=[]  SumI3OutMin=[]  SumI3OutMax=[]  SumI4OutMin=[]  SumI4OutMax=[]  SumDOutMin=[]  SumDOutMax=[]  DifferentiatorOutMin=[]  DifferentiatorOutMax=[]  FilterDiffOutCoefMin=[]  FilterDiffOutCoefMax=[]  ReciprocalOutMin=[]  ReciprocalOutMax=[]  SumDenOutMin=[]  SumDenOutMax=[]  SumNumOutMin=[]  SumNumOutMax=[]  DivideOutMin=[]  DivideOutMax=[]  UdiffTsProdOutMin=[]  UdiffTsProdOutMax=[]  NTsProdOutMin=[]  NTsProdOutMax=[]  UintegralTsProdOutMin=[]  UintegralTsProdOutMax=[]  UngainTsProdOutMin=[]  UngainTsProdOutMax=[]  ClampingZeroOutDataTypeStr=Inherit: Inherit via back propagation  ClampingZeroOutMin=[]  ClampingZeroOutMax=[]  FilterDenConstantOutDataTypeStr=Inherit: Inherit via back propagation  FilterDenConstantOutMin=[]  FilterDenConstantOutMax=[]  PCopyOutDataTypeStr=Inherit: Inherit via back propagation  PCopyOutMin=[]  PCopyOutMax=[]  NCopyOutDataTypeStr=Inherit: Inherit via back propagation  NCopyOutMin=[]  NCopyOutMax=[]  IntegratorContinuousStateAttributes=''  IntegratorStateMustResolveToSignalObject=off  IntegratorRTWStateStorageClass=Auto  FilterContinuousStateAttributes=''  FilterStateMustResolveToSignalObject=off  FilterRTWStateStorageClass=Auto  ParallelPVariant=InternalParameters  IdealPVariant=Disabled  IVariant=InternalParameters  DVariant=Disabled  IntegratorVariant=Continuous  SatVariant=Disabled  AWVariant=Passthrough  PCopyVariant=Disabled  TRVariant=Disabled  FdbkBlocksVariant=Forward  IdealPFdbkVariant=Disabled  SatFdbkVariant=Disabled  DerivativeFilterVariant=Disabled  NVariant=Disabled  NCopyVariant=Disabled_SignalSpec  FilterICVariant=Disabled  IntegratorICVariant=InternalICs  ExternalResetVariant=Disabled  TRSumVariant=Passthrough  SumFdbkVariant=Disabled  SumVariant=Sum_PI  TsampFilterVariant=InternalTs  TsampNgainVariant=Passthrough  TsampIntegralVariant=Disabled_SignalSpec  ExternalSaturationOutDataTypeStr=Inherit: Same as second input  DerivativeSourceVariant=Disabled
  Sum : Sum  Inputs=|+-
  PPfcmd : Outport
  SPfcmd : Outport  Port=2
  wires:
  Sum/1 -> PIu/1
  PIu/1 -> PPfcmd/1, SPfcmd/1
  u/1 -> Sum/2
  uRef/1 -> Sum/1

== system Drone2_simulink_old1/Hydrostatic & Hydrodynamic Effects/Added Mass Forces/Added Mass ==
  note: NOTE:
      | The forces due to added mass will me applied as external
      | forces, so they will oppose the direction of the accelerations
      |
      | $M_{rb}\dot{\nu}+C_{rb}(\nu)\nu= F_{propulsion} - M_a\dot{\nu}-C_a(\nu)\nu-D(\nu)\nu$
  Ma : Inport
  Abb : Inport  Port=2
  dwbdt : Inport  Port=3
  Demux : Demux  Outputs=[3,3]
  Gain : Gain  Gain=-1
  LPfilter : Subsystem
  Ma*[Abb,dwbdt]' : Product  Multiplication=Matrix(*)
  Reshape1 : Reshape  OutputDimensionality=Customize  OutputDimensions=[3,1]
  Reshape2 : Reshape  OutputDimensionality=Customize  OutputDimensions=[3,1]
  "[Abb,dwbdt]'" : Concatenate  Mode=Multidimensional array
  Fxyz : Outport
  Mxyz : Outport  Port=2
  wires:
  dwbdt/1 -> "[Abb,dwbdt]'"/2
  "[Abb,dwbdt]'"/1 -> Ma*[Abb,dwbdt]'/2
  Demux/2 -> Reshape2/1
  Ma/1 -> Ma*[Abb,dwbdt]'/1
  Abb/1 -> "[Abb,dwbdt]'"/1
  Demux/1 -> Reshape1/1
  Ma*[Abb,dwbdt]'/1 -> LPfilter/1(in)
  LPfilter/1(out) -> Gain/1
  Gain/1 -> Demux/1
  Reshape1/1 -> Fxyz/1
  Reshape2/1 -> Mxyz/1

== system Drone2_simulink_old1/Hydrostatic & Hydrodynamic Effects/Added Mass Forces/Coriolis ==
  note: Coriolis matrix
  note: NOTE:
      | It is important to mention that the coriolis matrix due to added mass
      | computed here includes the de-stabilizing Munk-moment .
      | This moment acts to turn the vehicle perpendicular to the flow, and it
      | is most dominant for slender body vehicles in pitch and yaw when the
      | lateral velocities are non-zero.
      | This de-stabilizing effect will need to be accounted for in the design
      | of the control algorithm.
  Vb : Inport
  wb : Inport  Port=2
  Ma : Inport  Port=3
  Ca(V) : Subsystem
  Ca(V)*[Vb,wb]' : Product  Multiplication=Matrix(*)
  Demux : Demux  Outputs=6
  Demux1 : Demux  Outputs=[3,3]
  Gain : Gain  Gain=-1
  Ma*[Vb,wb]' : Product  Multiplication=Matrix(*)
  "[Vb,wb]'" : Concatenate  Mode=Multidimensional array
  Fxyz : Outport
  Mxyz : Outport  Port=2
  wires:
  Ma/1 -> Ma*[Vb,wb]'/1
  Vb/1 -> "[Vb,wb]'"/1
  wb/1 -> "[Vb,wb]'"/2
  "[Vb,wb]'"/1 -> Ca(V)*[Vb,wb]'/2, Ma*[Vb,wb]'/2
  Ma*[Vb,wb]'/1 -> Demux/1
  Demux/1 -> Ca(V)/1(a1)  "a1"
  Demux/2 -> Ca(V)/2(a2)  "a2"
  Demux/3 -> Ca(V)/3(a3)  "a3"
  Demux/4 -> Ca(V)/4(b1)  "b1"
  Demux/5 -> Ca(V)/5(b2)  "b2"
  Demux/6 -> Ca(V)/6(b3)  "b3"
  Ca(V)/1(Ca(V)) -> Ca(V)*[Vb,wb]'/1
  Ca(V)*[Vb,wb]'/1 -> Gain/1
  Demux1/1 -> Fxyz/1
  Demux1/2 -> Mxyz/1
  Gain/1 -> Demux1/1

== system Drone2_simulink_old1/Hydrostatic & Hydrodynamic Effects/Drag Sub system/Aerodynamic drag ==
  Velocity : Inport
  Omega_b : Inport  Port=2
  Area : Subsystem
  Constant : Constant  Value=-Environment.Airdensity/2
  Linear drag : Constant  Value=diag([C_x C_y C_z])  mask{C_x=Vehicle.Air.Resistance.Cx, C_y=Vehicle.Air.Resistance.Cy, C_z=Vehicle.Air.Resistance.Cz}
      mask prompts: C_x "Drag X"; C_y "Drag Y"; C_z "Drag Z"
      mask DialogControl DescGroupVar Prompt: Drag
      mask DialogControl DescTextVar Prompt: Provide values for linear or rotation drage to formulate a diagonal  drag matrix
      mask Display: disp('diag([C_x C_y C_z])');
  MatrixMultiply{,1..3} (4 alike) : Product  Multiplication=Matrix(*)
  Reshape : Reshape  OutputDimensionality=Customize  OutputDimensions=[3,1]
  Reshape1 : Reshape  OutputDimensionality=Customize  OutputDimensions=[3,1]
  Rotational drag : Constant  Value=diag([C_x C_y C_z])  mask{C_x=Vehicle.Air.Resistance.Ck, C_y=Vehicle.Air.Resistance.Cm, C_z=Vehicle.Air.Resistance.Cn}
      mask prompts: C_x "Drag X"; C_y "Drag Y"; C_z "Drag Z"
      mask DialogControl DescGroupVar Prompt: Drag
      mask DialogControl DescTextVar Prompt: Provide values for linear or rotation drage to formulate a diagonal  drag matrix
      mask Display: disp('diag([C_x C_y C_z])');
  Subsystem : Subsystem
  Subsystem1 : Subsystem
  Force|_W : Outport
  Moment_W : Outport  Port=2
  wires:
  MatrixMultiply2/1 -> Force|_W/1
  Reshape1/1 -> MatrixMultiply3/2
  MatrixMultiply1/1 -> MatrixMultiply3/1
  Reshape/1 -> MatrixMultiply2/2
  MatrixMultiply/1 -> MatrixMultiply2/1
  Subsystem1/1(0.5rhov^2) -> Reshape1/1
  Area/2(Rotational) -> MatrixMultiply1/2
  Linear drag/1 -> MatrixMultiply/1
  Subsystem/1(0.5rhov^2) -> Reshape/1
  Rotational drag/1 -> MatrixMultiply1/1
  Area/1(Linear) -> MatrixMultiply/2
  Omega_b/1 -> Subsystem1/1(omega_b)
  Velocity/1 -> Subsystem/1(V_b)
  Constant/1 -> Subsystem1/2(rho), Subsystem/2(rho)
  MatrixMultiply3/1 -> Moment_W/1

== system Drone2_simulink_old1/Hydrostatic & Hydrodynamic Effects/Drag Sub system/Hydrodyanamic drag ==
  vr : Inport
  Omega_b : Inport  Port=2
  Area : Subsystem
  Constant : Constant  Value=-Environment.Waterdensity/2
  Linear drag : Constant  Value=diag([C_x C_y C_z])  mask{C_x=Vehicle.Water.Resistance.Cx, C_y=Vehicle.Water.Resistance.Cy, C_z=Vehicle.Water.Resistance.Cz}
      mask prompts: C_x "Drag X"; C_y "Drag Y"; C_z "Drag Z"
      mask DialogControl DescGroupVar Prompt: Drag
      mask DialogControl DescTextVar Prompt: Provide values for linear or rotation drage to formulate a diagonal  drag matrix
      mask Display: disp('diag([C_x C_y C_z])');
  MATLAB Function : MATLAB Function  TreatAsAtomicUnit=on  mask{MIN=-5, MAX=5}
  MATLAB Function1 : MATLAB Function  TreatAsAtomicUnit=on  mask{A=-0.1, B=0.1}
      mask prompts: A "Min"; B "Max"
  MatrixMultiply{,1..3} (4 alike) : Product  Multiplication=Matrix(*)
  Reshape : Reshape  OutputDimensionality=Customize  OutputDimensions=[3,1]
  Reshape1 : Reshape  OutputDimensionality=Customize  OutputDimensions=[3,1]
  Rotational drag : Constant  Value=diag([C_x C_y C_z])  mask{C_x=Vehicle.Water.Resistance.Ck, C_y=Vehicle.Water.Resistance.Cm, C_z=Vehicle.Water.Resistance.Cn}
      mask prompts: C_x "Drag X"; C_y "Drag Y"; C_z "Drag Z"
      mask DialogControl DescGroupVar Prompt: Drag
      mask DialogControl DescTextVar Prompt: Provide values for linear or rotation drage to formulate a diagonal  drag matrix
      mask Display: disp('diag([C_x C_y C_z])');
  Scope : Scope
  Subsystem : Subsystem
  Subsystem1 : Subsystem
  Force|_W : Outport
  Moment_W : Outport  Port=2
  wires:
  Constant/1 -> Subsystem1/2(rho), Subsystem/2(rho)
  vr/1 -> Subsystem/1(V_b)
  Omega_b/1 -> Subsystem1/1(omega_b)
  Area/1(Linear) -> MatrixMultiply/2
  Rotational drag/1 -> MatrixMultiply1/1
  Linear drag/1 -> MatrixMultiply/1
  Area/2(Rotational) -> MatrixMultiply1/2
  Subsystem1/1(0.5rhov^2) -> Reshape1/1
  MatrixMultiply/1 -> MatrixMultiply2/1
  Reshape/1 -> MatrixMultiply2/2
  MatrixMultiply1/1 -> MatrixMultiply3/1
  Reshape1/1 -> MatrixMultiply3/2
  MatrixMultiply2/1 -> MATLAB Function/1(u)
  MatrixMultiply3/1 -> MATLAB Function1/1(u)
  Subsystem/1(0.5rhov^2) -> Scope/1, Reshape/1
  MATLAB Function/1(y) -> Force|_W/1
  MATLAB Function1/1(y) -> Moment_W/1

== system Drone2_simulink_old1/Hydrostatic & Hydrodynamic Effects/Drag Sub system/Subsystem ==
  Altitude : Inport
  v : Inport  Port=2
  omega : Inport  Port=3
  Constant : Constant
  Subsystem : Subsystem
  Subsystem1 : Subsystem
  Subtract : Sum  Inputs=+-
  Transition Angular speed : Subsystem
  Transition data : Subsystem
  Transition speed : Subsystem
  1mwz : Outport
  W(z) : Outport  Port=2
  lambdav : Outport  Port=3
  lambdaomega : Outport  Port=4
  wires:
  Altitude/1 -> Transition data/1(Z)
  Subtract/1 -> 1mwz/1, Transition Angular speed/2(1mwz), Transition speed/2(1mwz)
  Constant/1 -> Subtract/1
  Transition data/1(W(z)) -> Subtract/2, W(z)/1, Transition Angular speed/1(W(z)), Transition speed/1(W(z))
  omega/1 -> Subsystem1/1(vector)
  Transition speed/1(lambdav) -> lambdav/1
  Transition Angular speed/1(lambdaomega) -> lambdaomega/1
  v/1 -> Subsystem/1(vector)
  Subsystem/1(Magnitude) -> Transition speed/3(vb)
  Subsystem1/1(Magnitude) -> Transition Angular speed/3(omegab)

== system Drone2_simulink_old1/Hydrostatic & Hydrodynamic Effects/Drag Sub system/Subsystem1 ==
  Vr : Inport
  omegab : Inport  Port=2
  Gain : Gain  Gain=0
  Linear drag : Constant  Value=diag([C_x C_y C_z])  mask{C_x=Vehicle.Water.LinearResistance.Cx, C_y=Vehicle.Water.LinearResistance.Cy, C_z=Vehicle.Water.LinearResistance.Cz}
      mask prompts: C_x "Drag X"; C_y "Drag Y"; C_z "Drag Z"
      mask DialogControl DescGroupVar Prompt: Drag
      mask DialogControl DescTextVar Prompt: Provide values for linear or rotation drage to formulate a diagonal  drag matrix
      mask Display: disp('diag([C_x C_y C_z])');
  Linear drag1 : Constant  Value=diag([C_x C_y C_z])  mask{C_x=Vehicle.Water.LinearResistance.Ck, C_y=Vehicle.Water.LinearResistance.Cm, C_z=Vehicle.Water.LinearResistance.Cn}
      mask prompts: C_x "Drag X"; C_y "Drag Y"; C_z "Drag Z"
      mask DialogControl DescGroupVar Prompt: Drag
      mask DialogControl DescTextVar Prompt: Provide values for linear or rotation drage to formulate a diagonal  drag matrix
      mask Display: disp('diag([C_x C_y C_z])');
  Product1 : Product  Multiplication=Matrix(*)
  Product3 : Product  Multiplication=Matrix(*)
  Saturation : Saturate  UpperLimit=1  LowerLimit=-1
  Saturation1 : Saturate  UpperLimit=5  LowerLimit=-5
  Scope : Scope  NumInputPorts=2
  linear drag : Outport
  linear wdrag : Outport  Port=2
  wires:
  Vr/1 -> Product3/2
  omegab/1 -> Product1/2
  Product1/1 -> Gain/1
  Linear drag/1 -> Product3/1
  Linear drag1/1 -> Product1/1
  Product3/1 -> Saturation1/1
  Saturation1/1 -> Scope/1, linear drag/1  "linear"
  Saturation/1 -> Scope/2, linear wdrag/1  "angular"
  Gain/1 -> Saturation/1

== system Drone2_simulink_old1/Hydrostatic & Hydrodynamic Effects/Ocean Current/Transition data ==
  Z : Inport
  Constant2 : Constant
  Exp : Math
  Gain : Gain  Gain=10/(Environment.Transition)
  Reciprocal : Product  Inputs=/
  Sum : Sum  Inputs=|++
  W(z) : Outport
  wires:
  Constant2/1 -> Sum/2
  Reciprocal/1 -> W(z)/1  "W(z)"
  Sum/1 -> Reciprocal/1
  Gain/1 -> Exp/1
  Z/1 -> Gain/1
  Exp/1 -> Sum/1

== system Drone2_simulink_old1/Hydrostatic & Hydrodynamic Effects/Wind force/Transition data ==
  Z : Inport
  Constant2 : Constant
  Exp : Math
  Gain : Gain  Gain=10/(Environment.Transition)
  Reciprocal : Product  Inputs=/
  Sum : Sum  Inputs=|++
  W(z) : Outport
  wires:
  Constant2/1 -> Sum/2
  Reciprocal/1 -> W(z)/1  "W(z)"
  Sum/1 -> Reciprocal/1
  Gain/1 -> Exp/1
  Z/1 -> Gain/1
  Exp/1 -> Sum/1
